simulink model "sim2"  (R2014a)
settings: Solver=ode45  StartTime=0.0  StopTime=24  RelTol=1e-3
values from neighbouring files (symbols this model uses):
  L1 = X1/(2*pi*f)    [machine2.m]
  L2 = X2/(2*pi*f)    [machine2.m]
  Lm = Lm*(a^2)    [machine2.m]
  R1 = (Req/2)*(a^2)    [machine2.m]
  R2 = Req/2    [machine2.m]
  Rc = Rc*(a^2)    [machine2.m]
  S = input('APPARENT POWER:')    [machine2.m]
  Vh = input('HIGH VOLTAGE:')    [machine2.m]
  Vl = input('LOW VOLTAGE:')    [machine2.m]
libraries: powerlib x18, dspstat3 x7, powerlib_meascontrol x2
settings Model: Creator=ASUS  LastModifiedBy=ASUS

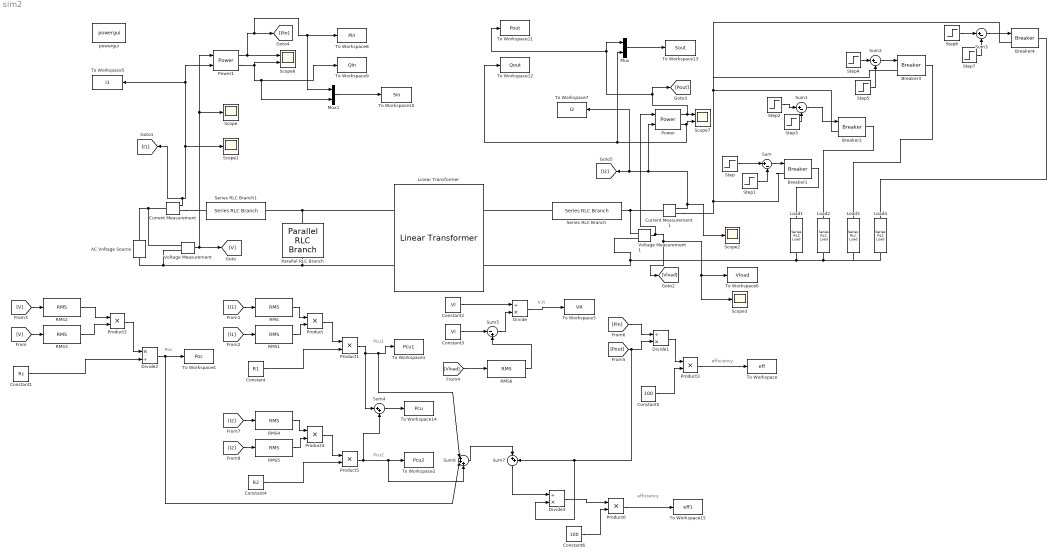
== system sim2 ==
  note: efficiency
  note: V.R
  note: Poc
  note: Pcu1
  note: Pcu2
  note: efficiency
  " Load1" : powerlib/Elements/Series RLC Load  LConnTagsString=a  RConnTagsString=__new0  NominalVoltage=Vl  NominalFrequency=50  ActivePower=0.3*S*0.8  InductivePower=0.3*S*0.6  CapacitivePower=0  Setx0=off  InitialVoltage=0  SetiL0=off  InitialCurrent=0  Measurements=None
  " Load2" : powerlib/Elements/Series RLC Load  LConnTagsString=a  RConnTagsString=__new0  NominalVoltage=Vl  NominalFrequency=50  ActivePower=0.75*S  InductivePower=0  CapacitivePower=0  Setx0=off  InitialVoltage=0  SetiL0=off  InitialCurrent=0  Measurements=None
  " Load3" : powerlib/Elements/Series RLC Load  LConnTagsString=a  RConnTagsString=__new0  NominalVoltage=Vl  NominalFrequency=50  ActivePower=S*0.9  InductivePower=S*0.44  CapacitivePower=0  Setx0=off  InitialVoltage=0  SetiL0=off  InitialCurrent=0  Measurements=None
  AC Voltage Source : powerlib/Electrical Sources/AC Voltage Source  Amplitude=Vh*(1.4142)  Phase=0  Frequency=50  SampleTime=0  Measurements=None
  "Breaker1 " : powerlib/Elements/Breaker  InitialState=0  SwitchingTimes="[1/60  5/60]"  External=on  BreakerResistance=0.01  SnubberResistance=1e6  SnubberCapacitance=inf  Measurements=None  MoreParameters=on  NoBreakLoop=off
  "Breaker2 " : powerlib/Elements/Breaker  InitialState=0  SwitchingTimes="[1/60  5/60]"  External=on  BreakerResistance=0.01  SnubberResistance=1e6  SnubberCapacitance=inf  Measurements=None  MoreParameters=on  NoBreakLoop=off
  "Breaker3 " : powerlib/Elements/Breaker  InitialState=0  SwitchingTimes="[1/60  5/60]"  External=on  BreakerResistance=0.01  SnubberResistance=1e6  SnubberCapacitance=inf  Measurements=None  MoreParameters=on  NoBreakLoop=off
  Breaker4 : powerlib/Elements/Breaker  InitialState=0  SwitchingTimes="[1/60  5/60]"  External=on  BreakerResistance=0.01  SnubberResistance=1e6  SnubberCapacitance=inf  Measurements=None  MoreParameters=on  NoBreakLoop=off
  Constant : Constant  Value=R1
  Constant1 : Constant  Value=Rc
  Constant2 : Constant  Value=Vl
  Constant3 : Constant  Value=Vl
  Constant4 : Constant  Value=R2
  Constant5 : Constant  Value=100
  Constant6 : Constant  Value=100
  Current Measurement : powerlib/Measurements/Current Measurement  PhasorSimulation=off  OutputType=Complex  PSBequivalent=0
  Current Measurement1 : powerlib/Measurements/Current Measurement  PhasorSimulation=off  OutputType=Complex  PSBequivalent=0
  Divide : Product  Inputs=/*
  Divide1 : Product  Inputs=/*
  Divide2 : Product  Inputs=*/
  Divide3 : Product  Inputs=/*
  Linear Transformer : powerlib/Elements/Linear Transformer  UNITS=SI  NominalPower=[S 50 ]  winding1=[Vh 0 0]  winding2=[Vl 0 0]  ThreeWindings=off  winding3=[3.15e+05 0.7938 0.084225]  RmLm=[2e+06 2e+06]  Measurements=None  DataType=on
  "Load4 " : powerlib/Elements/Series RLC Load  LConnTagsString=a  RConnTagsString=__new0  NominalVoltage=Vl  NominalFrequency=50  ActivePower=0.5*S*0.85  InductivePower=0.5*S*0.53  CapacitivePower=0  Setx0=off  InitialVoltage=0  SetiL0=off  InitialCurrent=0  Measurements=None
  Mux : Mux  Inputs=2
  Mux1 : Mux  Inputs=2
  Parallel RLC Branch : powerlib/Elements/Parallel RLC Branch  LConnTagsString=a  RConnTagsString=__new0  BranchType=RL  Resistance=Rc  Inductance=Lm  SetiL0=off  InitialCurrent=0  Capacitance=1e-6  Setx0=off  InitialVoltage=0  Measurements=None
  Power : powerlib_meascontrol/Measurements/Power  Freq=60  Vinit=[1, 0]  Iinit=[1, 0]  Ts=0
  Power1 : powerlib_meascontrol/Measurements/Power  Freq=60  Vinit=[1, 0]  Iinit=[1, 0]  Ts=0
  Product{,1..6} (7 alike) : Product
  RMS{,1..6} (7 alike) : dspstat3/RMS  run=off  reset_popup=None  InputProcessing=Columns as channels (frame based)  directionMode=Each column  dimension=1  treatSBRowAsCol=on
  Scope{,1..3} (4 alike) : Scope
      Scope settings: YMin=-4000  YMax=4000
      Scope2 settings: YMin=-10  YMax=10  SaveName=ScopeData2
      Scope3 settings: SaveName=ScopeData3
  Scope6 : Scope  NumInputPorts=2
      settings: YMin=-100~-5  YMax=150~5  SaveName=ScopeData6
  Scope7 : Scope  NumInputPorts=2
      settings: YMin=-1.5~-5  YMax=8~5  SaveName=ScopeData7
  Series RLC Branch : powerlib/Elements/Series RLC Branch  LConnTagsString=__new0  RConnTagsString=__new0  BranchType=RL  Resistance=R2  Inductance=L2  SetiL0=off  InitialCurrent=0  Capacitance=1e-6  Setx0=off  InitialVoltage=0  Measurements=None
  Series RLC Branch1 : powerlib/Elements/Series RLC Branch  LConnTagsString=__new0  RConnTagsString=__new0  BranchType=RL  Resistance=R1  Inductance=L1  SetiL0=off  InitialCurrent=0  Capacitance=1e-6  Setx0=off  InitialVoltage=0  Measurements=None
  Step : Step  Time=0  SampleTime=0
  Step1 : Step  Time=7  SampleTime=0
  Step2 : Step  Time=7  SampleTime=0
  Step3 : Step  Time=12  SampleTime=0
  Step4 : Step  Time=12  SampleTime=0
  Step5 : Step  Time=20  SampleTime=0
  Step6 : Step  Time=20  SampleTime=0
  Step7 : Step  Time=24  SampleTime=0
  Sum{,1..3} (4 alike) : Sum  Inputs=|+-
  Sum4 : Sum  Inputs=|++
  Sum5 : Sum  Inputs=|-+
  Sum6 : Sum  Inputs=|+++
  Sum7 : Sum  Inputs=|++
  To Workspace : ToWorkspace  VariableName=eff  SampleTime=-1
  To Workspace1 : ToWorkspace  VariableName=Pcu1  SampleTime=-1
  To Workspace10 : ToWorkspace  VariableName=Sin  SampleTime=-1
  To Workspace11 : ToWorkspace  VariableName=Pout  SampleTime=-1
  To Workspace12 : ToWorkspace  VariableName=Qout  SampleTime=-1
  To Workspace13 : ToWorkspace  VariableName=Sout  SampleTime=-1
  To Workspace14 : ToWorkspace  VariableName=Pcu  SampleTime=-1
  To Workspace15 : ToWorkspace  VariableName=eff1  SampleTime=-1
  To Workspace2 : ToWorkspace  VariableName=Pcu2  SampleTime=-1
  To Workspace3 : ToWorkspace  VariableName=VR  SampleTime=-1
  To Workspace4 : ToWorkspace  VariableName=Poc  SampleTime=-1
  To Workspace5 : ToWorkspace  VariableName=I1  SampleTime=-1
  To Workspace6 : ToWorkspace  VariableName=Vload  SampleTime=-1
  To Workspace7 : ToWorkspace  VariableName=I2  SampleTime=-1
  To Workspace8 : ToWorkspace  VariableName=Pin  SampleTime=-1
  To Workspace9 : ToWorkspace  VariableName=Qin  SampleTime=-1
  Voltage Measurement : powerlib/Measurements/Voltage Measurement  PhasorSimulation=off  OutputType=Complex  PSBequivalent=0
  Voltage Measurement1 : powerlib/Measurements/Voltage Measurement  PhasorSimulation=off  OutputType=Complex  PSBequivalent=0
  powergui : powerlib/powergui  Priority=1  SimulationMode=Discrete  SolverType=Tustin  SampleTime=50e-6  frequency=60  SPID=off  DisableSnubberDevices=off  DisableRonSwitches=off  DisableVfSwitches=off  SwTol=0  Interpol=off  DisplayEquations=off  Ts=0  methode=off  frequencyindice=50  Pbase=100e6  ErrMax=1e-4  Iterations=50  UnitsV=kV  UnitsW=MW  FunctionMessages=off  echomessages=off  HookPort=off  EnableUseOfTLC=off  x0status=blocks  RestoreLinks=warning  ResistiveCurrentMeasurement=off  Frange=[0:2:500]  Ylog=off  Xlog=on  ShowGrid=off  save=off  variable=ZData  structure=0  ZoomFFT=off  StartTime=0.0  cycles=1  DisplayStyle=1  fundamental=60  FreqAxis=off  MaxFrequency=1000  frequencyindicesteady=1  RmsSteady=1  display=off
  wires:
  Voltage Measurement/1 -> [V], Power1/1, Scope/1
  Step/1 -> Sum/1
  Step1/1 -> Sum/2
  Sum/1 -> "Breaker1 "/1
  Step2/1 -> Sum1/1
  Step3/1 -> Sum1/2
  Sum1/1 -> "Breaker2 "/1
  Step4/1 -> Sum2/1
  Step5/1 -> Sum2/2
  Sum2/1 -> "Breaker3 "/1
  Step6/1 -> Sum3/1
  Step7/1 -> Sum3/2
  Sum3/1 -> Breaker4/1
  Current Measurement/1 -> [I1], To Workspace5/1, Power1/2, Scope1/1
  Current Measurement1/1 -> Scope2/1, Power/2, To Workspace7/1, [I2]
  Voltage Measurement1/1 -> Power/1, To Workspace6/1, Scope3/1, [Vload]
  [I1] -> RMS/1
  [I1] -> RMS1/1
  RMS/1 -> Product/1
  RMS1/1 -> Product/2
  Constant/1 -> Product1/2
  Product/1 -> Product1/1
  [V] -> RMS2/1
  [V] -> RMS3/1
  RMS2/1 -> Product2/1
  RMS3/1 -> Product2/2
  Power1/2 -> Mux1/2, To Workspace9/1, Scope6/2
  Power1/1 -> Mux1/1, To Workspace8/1, [Pin], Scope6/1
  Power/1 -> Mux/1, To Workspace11/1, [Pout], Scope7/1
  Power/2 -> Mux/2, To Workspace12/1, Scope7/2
  Constant3/1 -> Sum5/1
  Constant2/1 -> Divide/1
  Sum5/1 -> Divide/2
  [Pout] -> Divide3/2, Sum7/2, Divide1/2
  [Pin] -> Divide1/1
  [I2] -> RMS4/1
  [I2] -> RMS5/1
  RMS4/1 -> Product4/1
  RMS5/1 -> Product4/2
  Constant4/1 -> Product5/2
  Product4/1 -> Product5/1
  Product1/1 -> Sum4/1, Sum6/1, To Workspace1/1
  Product5/1 -> Sum4/2, Sum6/3, To Workspace2/1
  Divide/1 -> To Workspace3/1
  Product2/1 -> Divide2/1
  Constant1/1 -> Divide2/2
  [Vload] -> RMS6/1
  RMS6/1 -> Sum5/2
  Divide2/1 -> Sum6/2, To Workspace4/1
  Constant5/1 -> Product3/2
  Divide1/1 -> Product3/1
  Product3/1 -> To Workspace/1
  Sum4/1 -> To Workspace14/1
  Sum6/1 -> Sum7/1
  Sum7/1 -> Divide3/1
  Constant6/1 -> Product6/2
  Product6/1 -> To Workspace15/1
  Divide3/1 -> Product6/1
  Mux1/1 -> To Workspace10/1
  Mux/1 -> To Workspace13/1
  connections:
  Voltage Measurement/LConn1 -- AC Voltage Source/RConn1 -- Current Measurement/LConn1
  Linear Transformer/LConn2 -- Voltage Measurement/LConn2 -- AC Voltage Source/LConn1 -- Parallel RLC Branch/RConn1
  Parallel RLC Branch/LConn1 -- Series RLC Branch1/RConn1 -- Linear Transformer/LConn1
  " Load1"/RConn1 -- " Load3"/RConn1 -- "Load4 "/RConn1 -- " Load2"/RConn1 -- Voltage Measurement1/LConn2 -- Linear Transformer/RConn2
  "Breaker1 "/LConn1 -- Current Measurement1/RConn1 -- "Breaker2 "/LConn1 -- "Breaker3 "/LConn1 -- Breaker4/LConn1
  "Breaker1 "/RConn1 -- " Load1"/LConn1
  "Breaker2 "/RConn1 -- " Load2"/LConn1
  "Breaker3 "/RConn1 -- " Load3"/LConn1
  "Load4 "/LConn1 -- Breaker4/RConn1
  Series RLC Branch/RConn1 -- Current Measurement1/LConn1 -- Voltage Measurement1/LConn1
  Current Measurement/RConn1 -- Series RLC Branch1/LConn1
  Series RLC Branch/LConn1 -- Linear Transformer/RConn1
